simulink model "GUI_SSB_F"  (R2020b)
settings: Solver=VariableStepAuto  StartTime=0.0  StopTime=10.0  RelTol=1e-3
undefined symbols (not defined in the file): carr, mssg
libraries: dsparch4 x1
settings Model: Creator=Satyam Morankar  LastModifiedBy=Satyam Morankar

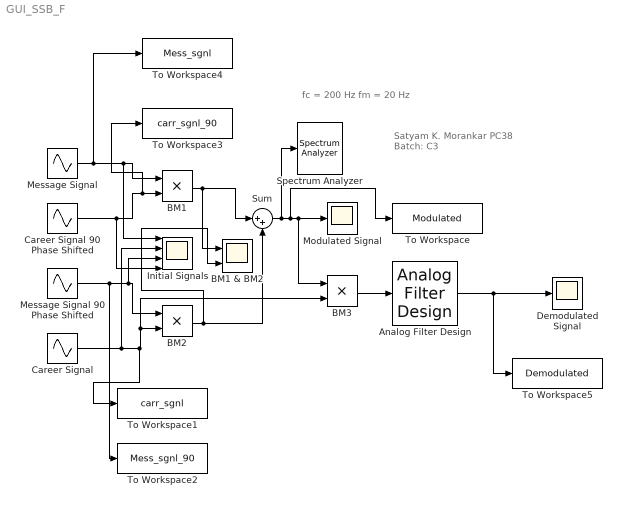
== system GUI_SSB_F ==
  note: Satyam K. Morankar
      | PC38
      | Batch: C3
  note: fc = 200 Hz
      | fm = 20 Hz
  Analog Filter Design : dsparch4/Analog Filter Design  method=Butterworth  filttype=Lowpass  N=8  Wlo=2*pi*mssg  Whi=80  Rp=2  Rs=40
  BM1 : Product
  BM1 & BM2 : Scope  NumInputPorts=2
  BM2 : Product
  BM3 : Product
  Career Signal : Sin  Frequency=2*pi*carr  SampleTime=1/5000
  Career Signal 90 Phase Shifted : Sin  Frequency=2*pi*carr  Phase=pi/2  SampleTime=1/5000
  Demodulated Signal : Scope
  Initial Signals : Scope  NumInputPorts=4
  Message Signal : Sin  Frequency=2*pi*mssg  SampleTime=1/5000
  Message Signal 90 Phase Shifted : Sin  Frequency=2*pi*mssg  Phase=pi/2  SampleTime=1/5000
  Modulated Signal : Scope
  Spectrum Analyzer : SpectrumAnalyzer
  Sum : Sum  Inputs=|++
  To Workspace : ToWorkspace  VariableName=Modulated  SaveFormat=Timeseries  SampleTime=-1
  To Workspace1 : ToWorkspace  VariableName=carr_sgnl  SaveFormat=Timeseries  SampleTime=-1
  To Workspace2 : ToWorkspace  VariableName=Mess_sgnl_90  SaveFormat=Timeseries  SampleTime=-1
  To Workspace3 : ToWorkspace  VariableName=carr_sgnl_90  SaveFormat=Timeseries  SampleTime=-1
  To Workspace4 : ToWorkspace  VariableName=Mess_sgnl  SaveFormat=Timeseries  SampleTime=-1
  To Workspace5 : ToWorkspace  VariableName=Demodulated  SaveFormat=Timeseries  SampleTime=-1
  wires:
  Sum/1 -> Spectrum Analyzer/1, To Workspace/1, BM3/1, Modulated Signal/1
  Career Signal 90 Phase Shifted/1 -> Initial Signals/4, To Workspace3/1, BM1/2
  BM3/1 -> Analog Filter Design/1
  Message Signal 90 Phase Shifted/1 -> To Workspace2/1, Initial Signals/3, BM2/1
  Message Signal/1 -> To Workspace4/1, Initial Signals/1, BM1/1
  BM2/1 -> Sum/2, BM1 & BM2/2
  Career Signal/1 -> Initial Signals/2, To Workspace1/1, BM2/2, BM3/2
  Analog Filter Design/1 -> To Workspace5/1, Demodulated Signal/1
  BM1/1 -> Sum/1, BM1 & BM2/1
